simulink model "Loops10"  (Simulink 6.0)
settings: Solver=ode45  StartTime=0.0  StopTime=10.0  RelTol=1e-3
settings Model: Creator=scaife  LastModifiedBy=scaife  ExtModeAutoUpdateStatusClock=off
settings DataIOCC: SignalLoggingName=sigsOut
settings DebuggingCC: SolverPrmCheckMsg=none
settings HardwareCC: TargetUnknown=on
settings GRTTargetCC: ModelReferenceCompliant=off  MatFileLogging=off

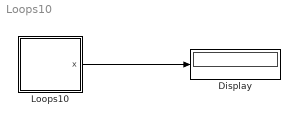
== system Loops10 ==
  Display : Display
  Loops10 : Stateflow chart
  wires:
  Loops10/1(x) -> Display/1

== stateflow chart Loops10 ==
  state A
  state B
  state C
  (default) -> A
  (junction 7) -> B : [x==0||x==2]
  (junction 6) -> C : [x==1]
  A -> (junction 8) : {x=0}
  C -> (junction 6) : {x=2}
  (junction 8) -> (junction 6) : [x==0||x==1]
  (junction 6) -> (junction 8) : [x==2||x==3]
  (junction 7) -> (junction 8) : [x==1]
  (junction 6) -> (junction 7) : [x==0]
  B -> (junction 7) : {x++}
  (junction 8) -> A : [x==3]
  (junction 8) -> (junction 7) : [x==2]
  (junction 7) -> (junction 6) : [x==3]
  data: x output int32
